simulink model "mRefTestModel"  (R2023b)
settings: Solver=VariableStepAuto  StartTime=0.0  StopTime=10.0  RelTol=1e-3
settings Model: Creator=neham  LastModifiedBy=neham

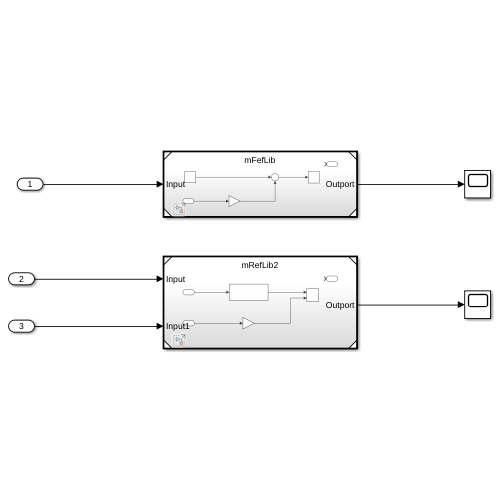
[thumbnail: Simulink's stored preview of the top-level diagram]
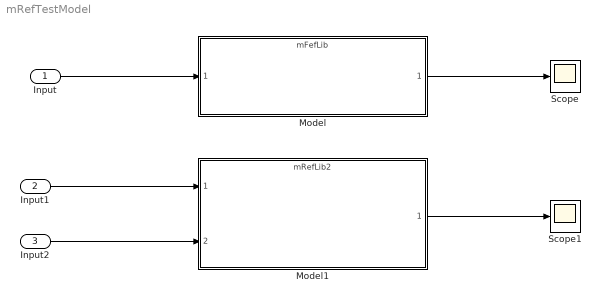
== system mRefTestModel ==
  Input : Inport
  Input1 : Inport  Port=2
  Input2 : Inport  Port=3
  Model : ModelReference  ModelNameDialog=mFefLib.slx  SimulationMode=Normal  ModelReferenceVersion=1.2
  Model1 : ModelReference  ModelNameDialog=mRefLib2.slx  SimulationMode=Normal  ModelReferenceVersion=1.2
  Scope : Scope
  Scope1 : Scope
  wires:
  Input/1 -> Model/1
  Input2/1 -> Model1/2
  Input1/1 -> Model1/1
  Model/1 -> Scope/1
  Model1/1 -> Scope1/1
